simulink model "modelo3"  (R2023b)
settings: Solver=ode45  StartTime=0  StopTime=10  FixedStep=1  RelTol=1e-3
undefined symbols (not defined in the file): ic_values, k_values, r_values
settings Model: Creator=anruk  LastModifiedBy=anruk

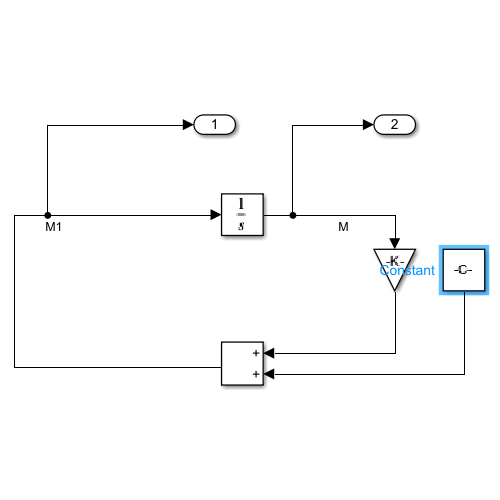
[thumbnail: Simulink's stored preview of the top-level diagram]
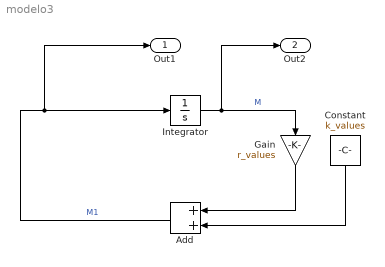
== system modelo3 ==
  Add : Sum
  Constant : Constant  Value=k_values
  Gain : Gain  Gain=r_values
  Integrator : Integrator  InitialCondition=ic_values(:,2)
  Out1 : Outport
  Out2 : Outport  Port=2
  wires:
  Add/1 -> Out1/1, Integrator/1  "M1"
  Integrator/1 -> Out2/1, Gain/1  "M"
  Gain/1 -> Add/1
  Constant/1 -> Add/2
